simulink model "LAB_2_simulink_LQR"  (R2022a)
settings: Solver=ode1  StartTime=0.0  StopTime=inf  FixedStep=0.002  RelTol=1e-3  EnableMultiTasking=on
PostLoadFcn:
  | qc_set_target_type(getConfigSet(bdroot, 'QUARC Default Target Configuration'));
values from neighbouring files (symbols this model uses):
  Joystick_gain_x = 1    [LAB_1_init.m]    (also in LAB_2_init_LQR.m; LAB_2_init_integral_LQR.m; LAB_3_init.m; LAB_4_init.m)
  Joystick_gain_y = -1    [LAB_1_init.m]    (also in LAB_2_init_LQR.m; LAB_2_init_integral_LQR.m; LAB_3_init.m; LAB_4_init.m)
  V_s0 = -(L_2/L_3)    (= 7.99069090909)    [LAB_1_init.m]    (also in LAB_2_init_LQR.m; LAB_2_init_integral_LQR.m; LAB_3_init.m; LAB_4_init.m)
undefined symbols (not defined in the file or in its folder): HIL, k_11, k_12, k_13, k_21, k_22, k_23, qc_get_step_size
libraries: quarc_library x4, simulink_extras x1
settings Model: SimulationMode=external  ExtModeTrigDuration=30000  Creator=Rchan  LastModifiedBy=Martynas
settings SolverCC: AlgebraicLoopSolver=TrustRegion  PositivePriorityOrder=on
settings DataIOCC: LimitDataPoints=on  SaveFormat=Array  SignalLoggingSaveFormat=ModelDataLogs  ReturnWorkspaceOutputs=off
settings OptimizationCC: ExpressionDepthLimit=2147483647  InitFltsAndDblsToZero=on  LifeSpan=inf
settings DebuggingCC: SaveWithParameterizedLinksMsg=none  UnderspecifiedInitializationDetection=Classic  MergeDetectMultiDrivingBlocksExec=none  SolverPrmCheckMsg=warning  MultiTaskDSMMsg=warning  MultiTaskCondExecSysMsg=none  FcnCallInpInsideContextMsg=warning  UnconnectedInputMsg=warning  UnconnectedOutputMsg=warning  UnconnectedLineMsg=warning  AllowSymbolicDim=off  StateNameClashWarn=warning  SFUnexpectedBacktrackingDiag=warning  SFNoUnconditionalDefaultTransitionDiag=warning  SFExecutionAtInitializationDiag=none  SFMachineParentedDataDiag=warning  ArithmeticOperatorsInVariantConditions=warning
settings HardwareCC: ProdBitPerPointer=32  ProdBitPerSizeT=32  ProdBitPerPtrDiffT=32  ProdLargestAtomicFloat=None  ProdIntDivRoundTo=Undefined  ProdEndianess=Unspecified  ProdWordSize=32  ProdHWDeviceType=32-bit Generic
settings ModelReferenceCC: PropagateSignalLabelsOutOfModel=off
settings SFSimCC: SimUseLocalCustomCode=off  CustomCodeUndefinedFunction=UseInterfaceOnly
settings RTWCC: Description=QUARC Win64 Target  SystemTargetFile=quarc_win64.tlc  TemplateMakefile=quarc_default_tmf  RTWUseLocalCustomCode=off  DLArmComputeVersion=19.05
settings CodeAppCC: StateflowObjectComments=on
settings STFCustomTargetCC: TargetPreCompLibLocation=C:\PROGRA~3\QUARC\lib\2020b\win64\release  ConcurrentExecutionCompliant=on  CPPClassGenCompliant=on  SystemTargetFile=quarc_win64.tlc
settings GRTTargetCC: TargetPreCompLibLocation=C:\PROGRA~3\QUARC\lib\2020b\win64\release  TargetLangStandard=C89/C90 (ANSI)  ParMdlRefBuildCompliant=off  CompOptLevelCompliant=off  CombineOutputUpdateFcns=off  MatFileLogging=off  GRTInterface=on  UseToolchainInfoCompliant=off  ExtMode=on  ExtModeMexFile=quarc_comm
settings ConfigComp: CovMetricSettings=dw  CovSaveCumulativeToWorkspaceVar=on  CovSaveSingleToWorkspaceVar=on  CovExternalEMLEnable=off  CovSFcnEnable=off

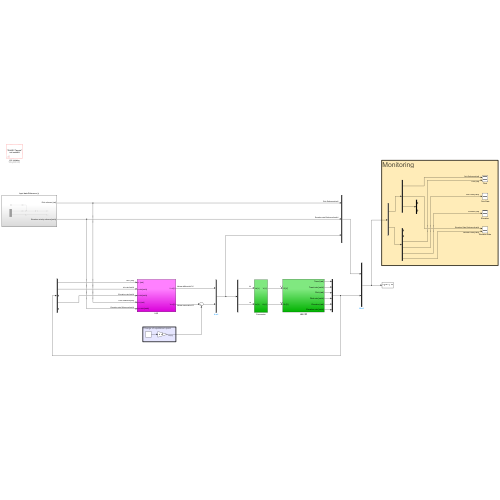
[thumbnail: Simulink's stored preview of the top-level diagram]
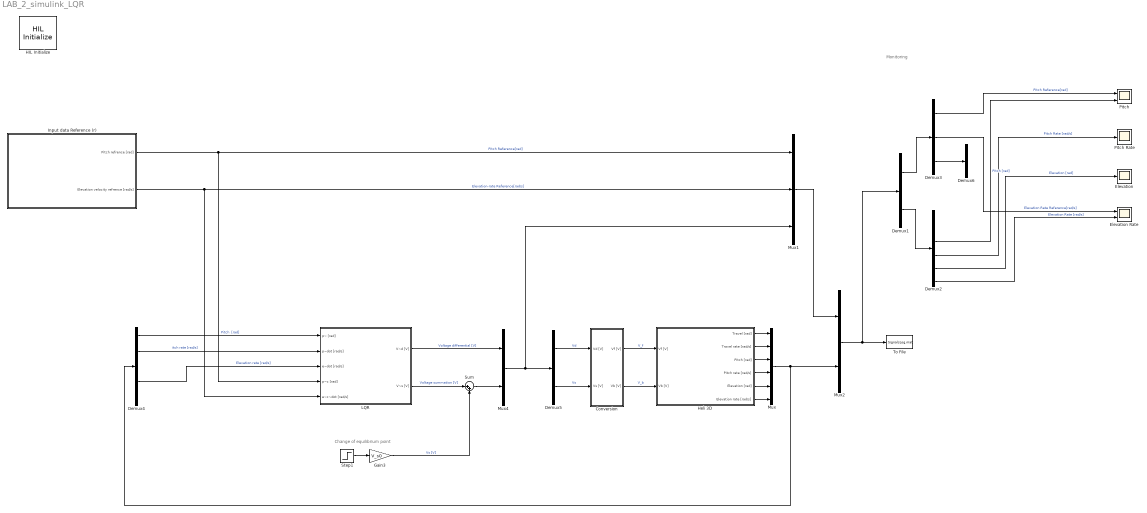
== system LAB_2_simulink_LQR ==
  note: Monitoring
  note: Change of equilibrium point
  Conversion : Subsystem
  Demux1 : Demux  Outputs=2
  Demux2 : Demux  Outputs=6
  Demux3 : Demux  Outputs=3
  Demux4 : Demux  Outputs=5
  Demux5 : Demux  Outputs=2
  Demux6 : Demux  Outputs=2
  Elevation : Scope
  Elevation Rate : Scope  NumInputPorts=2
  Gain3 : Gain  Gain=V_s0
  HIL Initialize : quarc_library/Data Acquisition/Generic/Configuration/HIL Initialize  Priority=-99  object_name=HIL-1  board_type=q8_usb  board_number=0  board_options=update_rate=normal;decimation=1  exclusive=off  active=off  hardware_clocks=[0:2]  clock_modes=[]  initial_clock_frequencies=[]  set_clock_params_at_start=off  set_clock_params_at_switch_in=off  set_clock_frequencies_at_start=off  set_clock_frequencies_at_switch_in=off  analog_input_channels=[0:7]  analog_input_configurations=[]  analog_input_maximums=10  analog_input_minimums=-10  set_analog_input_params_at_start=on  set_analog_input_params_at_switch_in=off  analog_output_channels=[0:7]  analog_output_maximums=10  analog_output_minimums=-10  initial_analog_outputs=[0]  final_analog_outputs=[0]  watchdog_analog_outputs=0  set_analog_output_params_at_start=on  set_analog_output_params_at_switch_in=off  set_analog_outputs_at_start=on  set_analog_outputs_at_switch_in=off  set_analog_outputs_at_terminate=on  set_analog_outputs_at_switch_out=off  set_analog_outputs_on_watchdog=off  digital_input_channels=[]  digital_output_channels=[]  digital_output_configuration=[]  initial_digital_outputs=[1]  final_digital_outputs=[1]  watchdog_digital_outputs=[1]  set_digital_output_params_at_start=off  set_digital_output_params_at_switch_in=off  set_digital_outputs_at_start=on  set_digital_outputs_at_switch_in=off  set_digital_outputs_at_terminate=on  set_digital_outputs_at_switch_out=off  set_digital_outputs_on_watchdog=off  encoder_channels=[0:7]  quadrature=[4]  encoder_filter_frequency=[]  initial_encoder_counts=[0]  set_encoder_params_at_start=on  set_encoder_params_at_switch_in=off  set_encoder_counts_at_start=on  set_encoder_counts_at_switch_in=off  pwm_channels=[0:7]  pwm_modes=0  pwm_frequency=99.532799999999995e6/4095  pwm_configuration=[0]  pwm_alignment=[0]  pwm_polarity=[1]  pwm_leading_deadband=[0]  pwm_trailing_deadband=[0]  initial_pwm_outputs=[0]  final_pwm_outputs=[0]  watchdog_pwm_outputs=[0]  set_pwm_params_at_start=on  set_pwm_params_at_switch_in=off  set_pwm_outputs_at_start=on  set_pwm_outputs_at_switch_in=off  set_pwm_outputs_at_terminate=on  set_pwm_outputs_at_switch_out=off  set_pwm_outputs_on_watchdog=off  other_output_channels=[]  initial_other_outputs=[]  final_other_outputs=[]  watchdog_other_outputs=[]  set_other_outputs_at_start=off  set_other_outputs_at_switch_in=off  set_other_outputs_at_terminate=off  set_other_outputs_at_switch_out=off  set_other_outputs_on_watchdog=off
  Heli 3D : Subsystem
  Input data Reference (r) : Subsystem
  LQR : Subsystem
  Mux : Mux  Inputs=6
  Mux1 : Mux  Inputs=3
  Mux2 : Mux  Inputs=2
  Mux4 : Mux  Inputs=2
  Pitch : Scope  NumInputPorts=2
  Pitch Rate : Scope
  Step1 : Step  SampleTime=0
  Sum : Sum  Inputs=|++
  To File : ToFile  Filename=SignalsLog.mat
  wires:
  Heli 3D/1(Travel [rad]) -> Mux/1
  Heli 3D/2(Travel rate [rad/s]) -> Mux/2
  Heli 3D/3(Pitch [rad]) -> Mux/3
  Heli 3D/4(Pitch rate [rad/s]) -> Mux/4
  Heli 3D/5(Elevation [rad]) -> Mux/5
  Heli 3D/6(Elevation rate [rad/s]) -> Mux/6
  Mux/1 -> Mux2/2, Demux4/1
  Demux4/1 -> LQR/1(p~ [rad])  "Pitch  [rad]"
  Demux4/2 -> LQR/2(p~dot [rad/s])  "itch rate [rad/s]"
  Demux4/4 -> LQR/3(e~dot [rad/s])  "Elevation rate [rad/s]"
  LQR/1(V~d [V]) -> Mux4/1  "Voltage differential [V]"
  Mux1/1 -> Mux2/1
  Mux2/1 -> Demux1/1, To File/1
  Gain3/1 -> Sum/2  "Vs [V]"
  Step1/1 -> Gain3/1
  LQR/2(V~s [V]) -> Sum/1  "Voltage summation [V]"
  Mux4/1 -> Mux1/3, Demux5/1
  Input data Reference (r)/1(Pitch refrence [rad]) -> LQR/4(p~c [rad]), Mux1/1  "Pitch Reference[rad]"
  Input data Reference (r)/2(Elevation velocity refrence [rad/s]) -> LQR/5(e~c~dot [rad/s]), Mux1/2  "Elevation-rate Reference[rad/s]"
  Sum/1 -> Mux4/2
  Demux5/2 -> Conversion/2(Vs [V])  "Vs"
  Demux5/1 -> Conversion/1(Vd [V])  "Vd"
  Conversion/1(Vf [V]) -> Heli 3D/1(Vf [V])  "V_f"
  Conversion/2(Vb [V]) -> Heli 3D/2(Vb [V])  "V_b"
  Demux1/1 -> Demux3/1
  Demux1/2 -> Demux2/1
  Demux3/3 -> Demux6/1
  Demux3/1 -> Pitch/1  "Pitch Reference[rad]"
  Demux3/2 -> Elevation Rate/1  "Elevation Rate Reference[rad/s]"
  Demux2/3 -> Pitch/2  "Pitch [rad]"
  Demux2/4 -> Pitch Rate/1  "Pitch Rate [rad/s]"
  Demux2/5 -> Elevation/1  "Elevation [rad]"
  Demux2/6 -> Elevation Rate/2  "Elevation Rate [rad/s]"

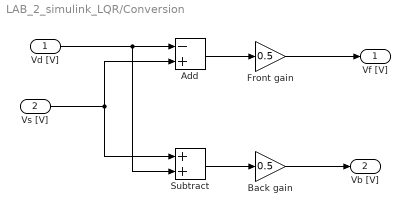
== system LAB_2_simulink_LQR/Conversion ==
  Vd [V] : Inport
  Vs [V] : Inport  Port=2
  Add : Sum  Inputs=-+
  Back gain : Gain  Gain=0.5
  Front gain : Gain  Gain=0.5
  Subtract : Sum
  Vf [V] : Outport
  Vb [V] : Outport  Port=2
  wires:
  Vd [V]/1 -> Subtract/2, Add/1
  Vs [V]/1 -> Subtract/1, Add/2
  Subtract/1 -> Back gain/1
  Back gain/1 -> Vb [V]/1
  Add/1 -> Front gain/1
  Front gain/1 -> Vf [V]/1

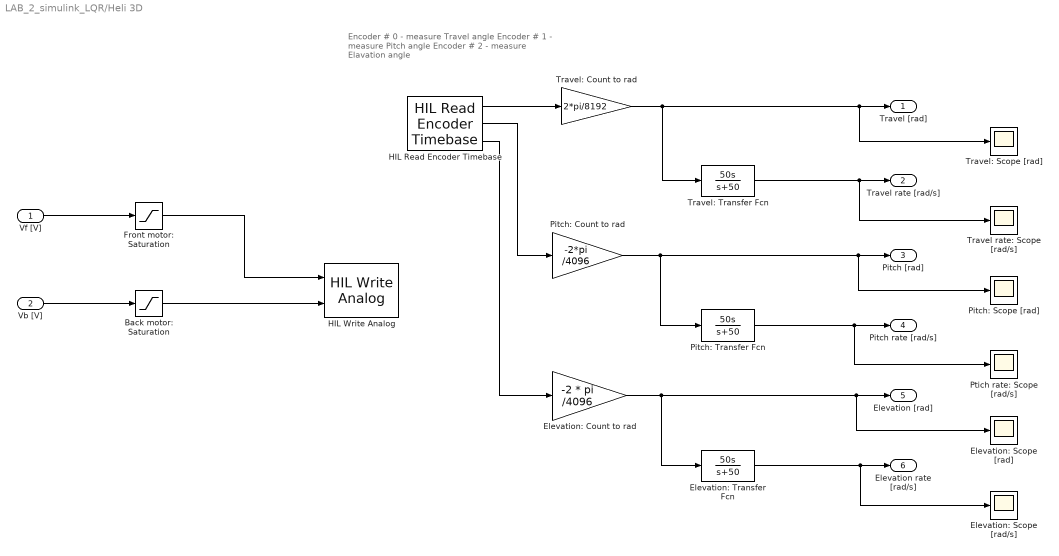
== system LAB_2_simulink_LQR/Heli 3D ==
  note: Encoder # 0 - measure Travel angle
      | Encoder # 1 - measure Pitch angle
      | Encoder # 2 - measure Elavation angle
  Vf [V] : Inport
  Vb [V] : Inport  Port=2
  Back motor: Saturation : Saturate  UpperLimit=5  LowerLimit=-5
  Elevation: Count to rad : Gain  Gain=-2 * pi /4096
  Elevation: Scope [rad/s] : Scope
  Elevation: Scope [rad] : Scope
  Elevation: Transfer Fcn : TransferFcn  Numerator=[50 0]  Denominator=[1 50]
  Front motor: Saturation : Saturate  UpperLimit=5  LowerLimit=-5
  HIL Read Encoder Timebase : quarc_library/Data Acquisition/Generic/Timebases/HIL Read Encoder Timebase  object_name=HIL-1  clock=0  channels=[0:2]  active=on  vector_output=off  data_type_mode=Inherit via back propagation  data_type=double  overflow_mode=Error on overflow  samples_in_buffer=max(ceil(1/qc_get_step_size), 1)
  HIL Write Analog : quarc_library/Data Acquisition/Generic/Immediate I//O/HIL Write Analog  object_name=HIL-1  channels=[0:1]  sample_time=-1  active=off  vector_input=off
  Pitch: Count to rad : Gain  Gain=-2*pi /4096
  Pitch: Scope [rad] : Scope
  Pitch: Transfer Fcn : TransferFcn  Numerator=[50 0]  Denominator=[1 50]
  Ptich rate: Scope [rad/s] : Scope
  Travel rate: Scope [rad/s] : Scope
  Travel: Count to rad : Gain  Gain=2*pi/8192
  Travel: Scope [rad] : Scope
  Travel: Transfer Fcn : TransferFcn  Numerator=[50 0]  Denominator=[1 50]
  Travel [rad] : Outport
  Travel rate [rad/s] : Outport  Port=2
  Pitch [rad] : Outport  Port=3
  Pitch rate [rad/s] : Outport  Port=4
  Elevation [rad] : Outport  Port=5
  Elevation rate [rad/s] : Outport  Port=6
  wires:
  HIL Read Encoder Timebase/1 -> Travel: Count to rad/1
  HIL Read Encoder Timebase/2 -> Pitch: Count to rad/1
  HIL Read Encoder Timebase/3 -> Elevation: Count to rad/1
  Travel: Count to rad/1 -> Travel: Scope [rad]/1, Travel [rad]/1, Travel: Transfer Fcn/1
  Travel: Transfer Fcn/1 -> Travel rate: Scope [rad/s]/1, Travel rate [rad/s]/1
  Pitch: Count to rad/1 -> Pitch: Transfer Fcn/1, Pitch: Scope [rad]/1, Pitch [rad]/1
  Pitch: Transfer Fcn/1 -> Ptich rate: Scope [rad/s]/1, Pitch rate [rad/s]/1
  Elevation: Count to rad/1 -> Elevation: Transfer Fcn/1, Elevation: Scope [rad]/1, Elevation [rad]/1
  Elevation: Transfer Fcn/1 -> Elevation: Scope [rad/s]/1, Elevation rate [rad/s]/1
  Vf [V]/1 -> Front motor: Saturation/1
  Vb [V]/1 -> Back motor: Saturation/1
  Front motor: Saturation/1 -> HIL Write Analog/1
  Back motor: Saturation/1 -> HIL Write Analog/2

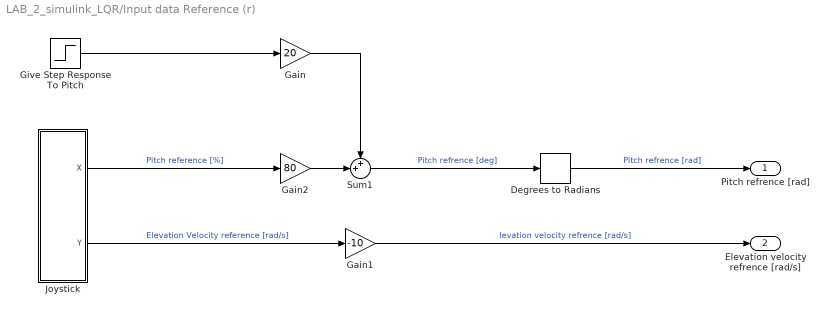
== system LAB_2_simulink_LQR/Input data Reference (r) ==
  Degrees to Radians : simulink_extras/Transformations/Degrees to Radians
  Gain : Gain  Gain=20
  Gain1 : Gain  Gain=-10
  Gain2 : Gain  Gain=80
  Give Step Response To Pitch : Step  Time=15  SampleTime=0
  Joystick : Subsystem
  Sum1 : Sum  Inputs=++|
  Pitch refrence [rad] : Outport
  Elevation velocity refrence [rad/s] : Outport  Port=2
  wires:
  Gain1/1 -> Elevation velocity refrence [rad/s]/1  "levation velocity refrence [rad/s]"
  Degrees to Radians/1 -> Pitch refrence [rad]/1  "Pitch refrence [rad]"
  Gain2/1 -> Sum1/2
  Give Step Response To Pitch/1 -> Gain/1
  Sum1/1 -> Degrees to Radians/1  "Pitch refrence [deg]"
  Gain/1 -> Sum1/1
  Joystick/1(X) -> Gain2/1  "Pitch reference [%]"
  Joystick/2(Y) -> Gain1/1  "Elevation Velocity reference [rad/s]"

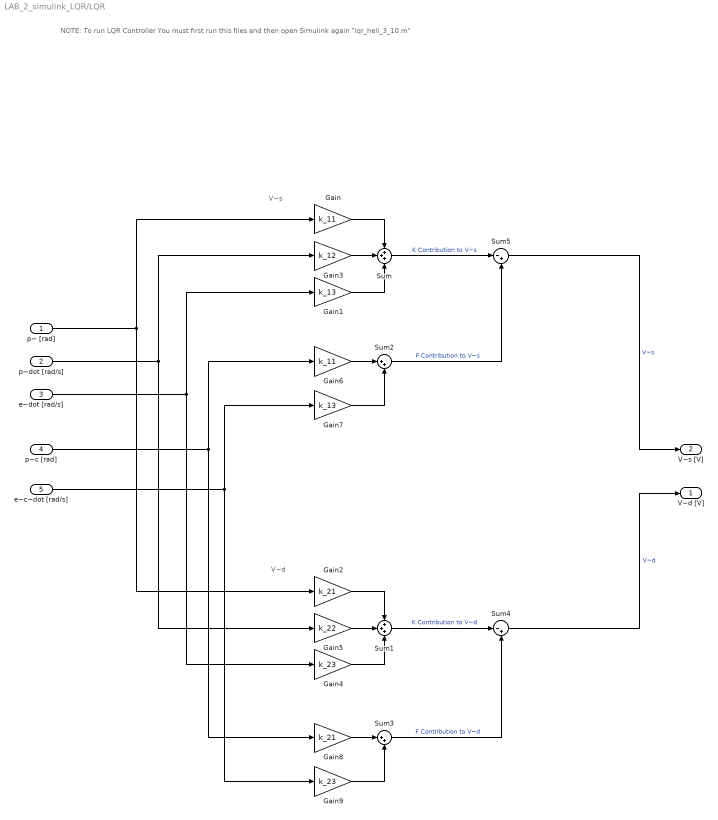
== system LAB_2_simulink_LQR/LQR ==
  note: NOTE: To run LQR Controller
      | You must first run this files and then open Simulink again
      | "lqr_heli_3_10.m"
  note: V~d
  note: V~s
  p~ [rad] : Inport
  p~dot [rad/s] : Inport  Port=2
  e~dot [rad/s] : Inport  Port=3
  p~c [rad] : Inport  Port=4
  e~c~dot [rad/s] : Inport  Port=5
  Gain : Gain  Gain=k_11
  Gain1 : Gain  Gain=k_13
  Gain2 : Gain  Gain=k_21
  Gain3 : Gain  Gain=k_12
  Gain4 : Gain  Gain=k_23
  Gain5 : Gain  Gain=k_22
  Gain6 : Gain  Gain=k_11
  Gain7 : Gain  Gain=k_13
  Gain8 : Gain  Gain=k_21
  Gain9 : Gain  Gain=k_23
  Sum : Sum  Inputs=+++
  Sum1 : Sum  Inputs=+++
  Sum2 : Sum  Inputs=|++
  Sum3 : Sum  Inputs=|++
  Sum4 : Sum  Inputs=|-+
  Sum5 : Sum  Inputs=|-+
  V~d [V] : Outport  InitialOutput=0
  V~s [V] : Outport  Port=2  InitialOutput=0
  wires:
  p~dot [rad/s]/1 -> Gain5/1, Gain3/1
  e~dot [rad/s]/1 -> Gain4/1, Gain1/1
  Gain/1 -> Sum/1
  Gain3/1 -> Sum/2
  Gain1/1 -> Sum/3
  p~ [rad]/1 -> Gain2/1, Gain/1
  Gain5/1 -> Sum1/2
  Gain2/1 -> Sum1/1
  Gain4/1 -> Sum1/3
  p~c [rad]/1 -> Gain6/1, Gain8/1
  e~c~dot [rad/s]/1 -> Gain7/1, Gain9/1
  Gain6/1 -> Sum2/1
  Gain7/1 -> Sum2/2
  Gain9/1 -> Sum3/2
  Gain8/1 -> Sum3/1
  Sum3/1 -> Sum4/2  "F Contribution to V~d"
  Sum1/1 -> Sum4/1  "K Contribution to V~d"
  Sum/1 -> Sum5/1  "K Contribution to V~s"
  Sum2/1 -> Sum5/2  "F Contribution to V~s"
  Sum5/1 -> V~s [V]/1  "V~s"
  Sum4/1 -> V~d [V]/1  "V~d"

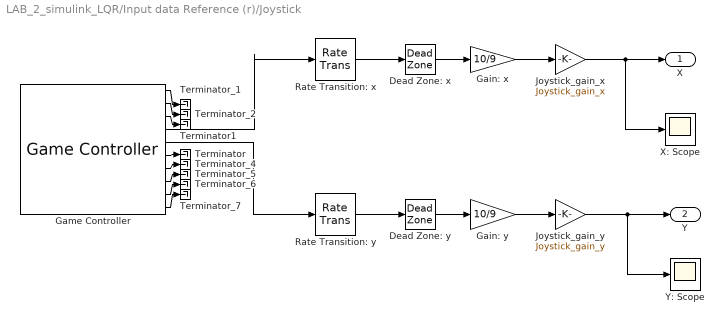
== system LAB_2_simulink_LQR/Input data Reference (r)/Joystick ==
  Dead Zone: x : DeadZone  LowerValue=-0.1  UpperValue=0.1
  Dead Zone: y : DeadZone  LowerValue=-0.1  UpperValue=0.1
  Gain: x : Gain  Gain=10/9
  Gain: y : Gain  Gain=10/9
  Game Controller : quarc_library/Devices/Peripherals/Target/Game Controller  controller=1  buffer_size=12  deadzone=[]  saturation=[]  sample_time=max(qc_get_step_size, 0.01)  auto_center=off  enabled=on
      settings: SourceProductName=QUARC Targets
  Joystick_gain_x : Gain  Gain=Joystick_gain_x
  Joystick_gain_y : Gain  Gain=Joystick_gain_y
  Rate Transition: x : RateTransition
  Rate Transition: y : RateTransition
  Terminator : Terminator
  Terminator1 : Terminator
  Terminator_{1..2,4..7} (6 alike) : Terminator
  X: Scope : Scope
  Y: Scope : Scope
  X : Outport
  Y : Outport  Port=2
  wires:
  Rate Transition: y/1 -> Dead Zone: y/1
  Rate Transition: x/1 -> Dead Zone: x/1
  Game Controller/5 -> Rate Transition: y/1
  Game Controller/4 -> Rate Transition: x/1
  Game Controller/1 -> Terminator_1/1
  Game Controller/2 -> Terminator_2/1
  Game Controller/7 -> Terminator_4/1
  Game Controller/8 -> Terminator_5/1
  Game Controller/9 -> Terminator_6/1
  Game Controller/10 -> Terminator_7/1
  Game Controller/3 -> Terminator1/1
  Game Controller/6 -> Terminator/1
  Dead Zone: x/1 -> Gain: x/1
  Dead Zone: y/1 -> Gain: y/1
  Gain: x/1 -> Joystick_gain_x/1
  Gain: y/1 -> Joystick_gain_y/1
  Joystick_gain_x/1 -> X/1, X: Scope/1
  Joystick_gain_y/1 -> Y: Scope/1, Y/1
